simulink model "model4_Linmod"  (R2021a)
settings: Solver=VariableStepAuto  StartTime=0.0  StopTime=10.0  MaxStep=1e-4  RelTol=1e-3
undefined symbols (not defined in the file): D, K1, K2, m1, m2
settings Model: Creator=Luka  LastModifiedBy=Luka

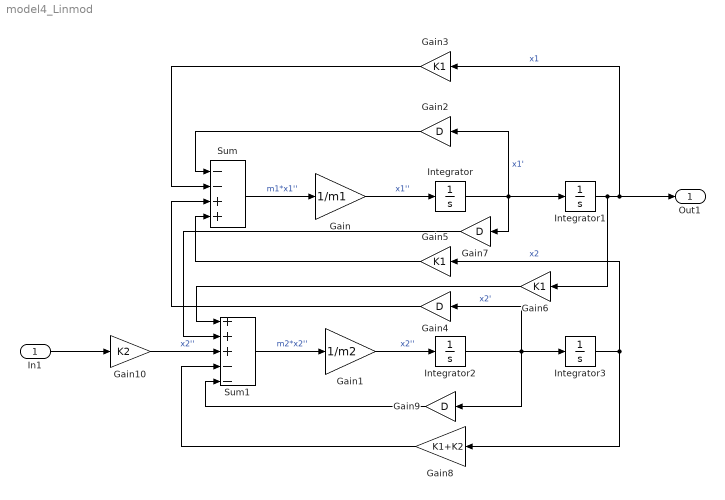
== system model4_Linmod ==
  In1 : Inport
  Gain : Gain  Gain=1/m1
  Gain1 : Gain  Gain=1/m2
  Gain10 : Gain  Gain=K2
  Gain{2,4,7,9} (4 alike) : Gain  Gain=D
  Gain3 : Gain  Gain=K1
  Gain5 : Gain  Gain=K1
  Gain6 : Gain  Gain=K1
  Gain8 : Gain  Gain=K1+K2
  Integrator{,1..3} (4 alike) : Integrator
  Sum : Sum  Inputs=--++
  Sum1 : Sum  Inputs=+++--
  Out1 : Outport
  wires:
  Integrator/1 -> Gain7/1, Gain2/1, Integrator1/1  "x1'"
  Integrator2/1 -> Gain4/1, Gain9/1, Integrator3/1  "x2'"
  Integrator1/1 -> Out1/1, Gain3/1, Gain6/1  "x1"
  Integrator3/1 -> Gain8/1, Gain5/1  "x2"
  Gain/1 -> Integrator/1  "x1''"
  Sum/1 -> Gain/1  "m1*x1''"
  Sum1/1 -> Gain1/1  "m2*x2''"
  Gain1/1 -> Integrator2/1  "x2''"
  Gain2/1 -> Sum/1
  Gain3/1 -> Sum/2
  Gain5/1 -> Sum/4
  Gain4/1 -> Sum/3
  Gain6/1 -> Sum1/1
  Gain7/1 -> Sum1/2
  Gain9/1 -> Sum1/5
  Gain8/1 -> Sum1/4
  Gain10/1 -> Sum1/3  "x2''"
  In1/1 -> Gain10/1
